simulink model "three_phase_voltage_drop_with_compensation"  (R2024a)
settings: Solver=VariableStepAuto  StartTime=0.0  StopTime=0.4  RelTol=1e-3
undefined symbols (not defined in the file): f, L_line, Q_cap, R_line, V_ll
libraries: dspstat3 x3, spsThreePhaseVIMeasurementLib x2, spsPower3phInstantaneousLib x1, spsThreePhaseParallelRLCLoadLib x1, spsThreePhaseSeriesRLCBranchLib x1, spsThreePhaseSeriesRLCLoadLib x1, spsThreePhaseSourceLib x1, spspowerguiLib x1
settings Model: Creator=m2  LastModifiedBy=m2

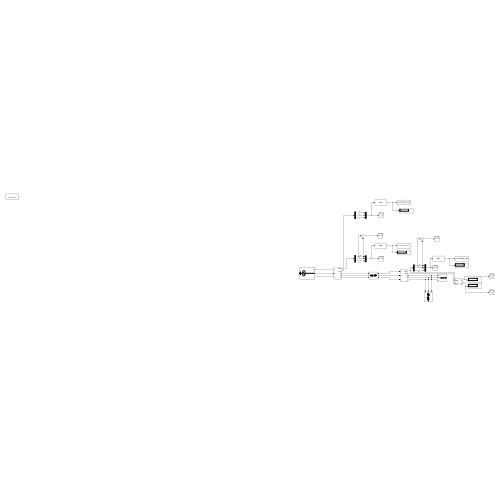
[thumbnail: Simulink's stored preview of the top-level diagram]
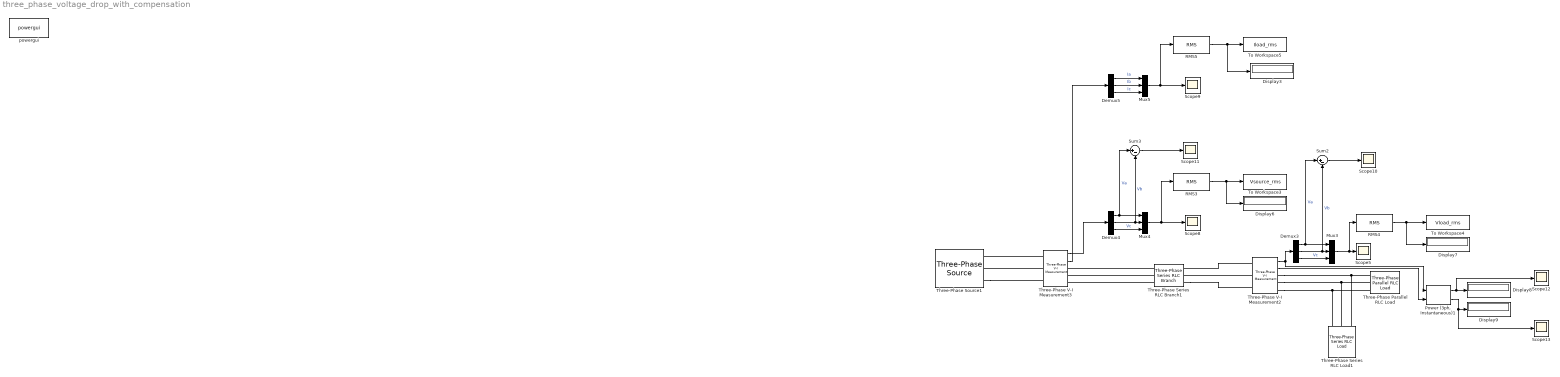
== system three_phase_voltage_drop_with_compensation ==
  Demux3 : Demux  Outputs=3
  Demux4 : Demux  Outputs=3
  Demux5 : Demux  Outputs=3
  Display{3,6..9} (5 alike) : Display
  Mux3 : Mux  Inputs=3
  Mux4 : Mux  Inputs=3
  Mux5 : Mux  Inputs=3
  "Power (3ph, Instantaneous)1" : spsPower3phInstantaneousLib/Power (3ph, Instantaneous)
  RMS3 : dspstat3/RMS  run=off  directionMode=Each column  dimension=1  InputProcessing=Columns as channels (frame based)  reset_popup=None
  RMS4 : dspstat3/RMS  run=off  directionMode=Each column  dimension=1  InputProcessing=Columns as channels (frame based)  reset_popup=None
  RMS5 : dspstat3/RMS  run=off  directionMode=Each column  dimension=1  InputProcessing=Columns as channels (frame based)  reset_popup=None
  Scope{5,8..13} (7 alike) : Scope
  Sum2 : Sum  Inputs=|+-
  Sum3 : Sum  Inputs=|+-
  Three-Phase Parallel RLC Load : spsThreePhaseParallelRLCLoadLib/Three-Phase Parallel RLC Load  LConnTagsString=A|B|C  Configuration=Y (grounded)  NominalVoltage=V_ll  Vabc=[1e3 1e3 1e3]  Vabcp=[1e3 1e3 1e3]  NominalFrequency=f  UnbalancedPower=off  ActivePower=0  InductivePower=0  CapacitivePower=-Q_cap  Pabc=[10e3 9e3 11e3]  QLabc=[100 90 110]  QCabc=[100 90 110]  Pabcp=[10e3 9e3 11e3]  QLabcp=[100 90 110]  QCabcp=[100 90 110]  Measurements=None  LoadType=constant Z
  Three-Phase Series RLC Branch1 : spsThreePhaseSeriesRLCBranchLib/Three-Phase Series RLC Branch  LConnTagsString=A|B|C  RConnTagsString=A|B|C  BranchType=RL  Resistance=R_line  Inductance=L_line  Capacitance=1e-6  Measurements=None
  Three-Phase Series RLC Load1 : spsThreePhaseSeriesRLCLoadLib/Three-Phase Series RLC Load  LConnTagsString=A|B|C  Configuration=Y (grounded)  NominalVoltage=400  Vabc=[1e3 1e3 1e3]  Vabcp=[1e3 1e3 1e3]  NominalFrequency=f  UnbalancedPower=off  ActivePower=P_load  InductivePower=Q_load  CapacitivePower=0  Pabc=[10e3 9e3 11e3]  QLabc=[100 90 110]  QCabc=[100 90 110]  Pabcp=[10e3 9e3 11e3]  QLabcp=[100 90 110]  QCabcp=[100 90 110]  Measurements=None  LoadType=constant Z
  Three-Phase V-I Measurement2 : spsThreePhaseVIMeasurementLib/Three-Phase V-I Measurement  VoltageMeasurement=phase-to-ground  SetLabelV=off  LabelV=Vabc  Vpu=off  VpuLL=off  CurrentMeasurement=yes  SetLabelI=off  LabelI=Iabc  Ipu=off  Pbase=100e6  Vbase=500e3  OutputType=Complex  PhasorSimulation=off  PSBequivalent=0
  Three-Phase V-I Measurement3 : spsThreePhaseVIMeasurementLib/Three-Phase V-I Measurement  VoltageMeasurement=phase-to-ground  SetLabelV=off  LabelV=Vabc  Vpu=off  VpuLL=off  CurrentMeasurement=yes  SetLabelI=off  LabelI=Iabc  Ipu=off  Pbase=100e6  Vbase=500e3  OutputType=Complex  PhasorSimulation=off  PSBequivalent=0
  Three-Phase Source1 : spsThreePhaseSourceLib/Three-Phase Source  InternalConnection=Yg  VoltagePhases=off  Voltage=V_ll  PhaseAngle=0  Voltage_phases=[25e3 25e3 25e3]/sqrt(3)  PhaseAngles_phases=[0 -120 +120]  Frequency=f  NonIdealSource=off  SpecifyImpedance=off  Resistance=0.8929  Inductance=16.58e-3  ShortCircuitLevel=100e6  BaseVoltage=25e3  XRratio=7  BusType=swing  Pref=10e3  Qref=0  Prefabc=[10e3, 10e3, 10e3]  Qrefabc=[0, 0, 0]  Qmin=-inf  Qmax=inf
  To Workspace3 : ToWorkspace  VariableName=Vsource_rms  SaveFormat=Timeseries  SampleTime=-1
  To Workspace4 : ToWorkspace  VariableName=Vload_rms  SaveFormat=Timeseries  SampleTime=-1
  To Workspace5 : ToWorkspace  VariableName=Iload_rms  SaveFormat=Timeseries  SampleTime=-1
  powergui : spspowerguiLib/powergui  Priority=1  SimulationMode=Continuous  SampleTime=50e-6  frequency=60  Iterations=50  frequencyindice=50  Pbase=100e6  ErrMax=1e-4  UnitsV=kV  UnitsW=MW  buscounter=0  FunctionMessages=off  echomessages=off  EnableUseOfTLC=off  CurrentSourceSwitches=off  DisableSnubberDevices=off  DisableRonSwitches=off  DisableVfSwitches=off  DisplayEquations=off  AutomaticDiscreteSolvers=off  SolverType=Tustin/Backward Euler (TBE)  Interpol=off  ExternalGateDelay=off  methode=off  Ts=100  x0status=blocks  SPID=on  SwTol=0  HookPort=off  NonlinearTolerance=1e-4  nMaxIteration=100  ContinueOnMaxIteration=off  RestoreLinks=warning  ResistiveCurrentMeasurement=off  Frange=[0:2:500]  Ylog=off  Xlog=on  ShowGrid=off  save=off  variable=ZData  structure=0  ZoomFFT=off  StartTime=0.0  cycles=1  DisplayStyle=1  fundamental=60  FreqAxis=off  MaxFrequency=1000  frequencyindicesteady=1  RmsSteady=1  display=off
  wires:
  Sum2/1 -> Scope10/1
  RMS5/1 -> Display3/1, To Workspace5/1
  Demux4/1 -> Sum3/1, Mux4/1  "Va"
  Demux4/2 -> Sum3/2, Mux4/2  "Vb"
  Three-Phase V-I Measurement2/2 -> "Power (3ph, Instantaneous)1"/2
  "Power (3ph, Instantaneous)1"/2 -> Scope13/1, Display9/1
  Demux5/3 -> Mux5/3  "Ic"
  RMS4/1 -> To Workspace4/1, Display7/1
  Mux5/1 -> RMS5/1, Scope9/1
  Mux4/1 -> RMS3/1, Scope8/1
  Three-Phase V-I Measurement3/1 -> Demux4/1
  Three-Phase V-I Measurement3/2 -> Demux5/1
  Demux3/3 -> Mux3/3  "Vc"
  Demux5/1 -> Mux5/1  "Ia"
  Demux3/2 -> Sum2/2, Mux3/2  "Vb"
  "Power (3ph, Instantaneous)1"/1 -> Scope12/1, Display8/1
  Demux4/3 -> Mux4/3  "Vc"
  RMS3/1 -> Display6/1, To Workspace3/1
  Mux3/1 -> RMS4/1, Scope5/1
  Three-Phase V-I Measurement2/1 -> "Power (3ph, Instantaneous)1"/1, Demux3/1
  Demux5/2 -> Mux5/2  "Ib"
  Sum3/1 -> Scope11/1
  Demux3/1 -> Sum2/1, Mux3/1  "Va"
  connections:
  Three-Phase Series RLC Branch1/LConn2 -- Three-Phase V-I Measurement3/RConn2
  Three-Phase V-I Measurement2/RConn1 -- Three-Phase Parallel RLC Load/LConn1 -- Three-Phase Series RLC Load1/LConn3
  Three-Phase V-I Measurement2/RConn2 -- Three-Phase Series RLC Load1/LConn2 -- Three-Phase Parallel RLC Load/LConn2
  Three-Phase Series RLC Branch1/RConn3 -- Three-Phase V-I Measurement2/LConn3
  Three-Phase V-I Measurement2/LConn1 -- Three-Phase Series RLC Branch1/RConn1
  Three-Phase Series RLC Branch1/LConn1 -- Three-Phase V-I Measurement3/RConn1
  Three-Phase V-I Measurement2/LConn2 -- Three-Phase Series RLC Branch1/RConn2
  Three-Phase V-I Measurement3/LConn1 -- Three-Phase Source1/RConn1
  Three-Phase Series RLC Branch1/LConn3 -- Three-Phase V-I Measurement3/RConn3
  Three-Phase V-I Measurement2/RConn3 -- Three-Phase Parallel RLC Load/LConn3 -- Three-Phase Series RLC Load1/LConn1
  Three-Phase Source1/RConn3 -- Three-Phase V-I Measurement3/LConn3
  Three-Phase V-I Measurement3/LConn2 -- Three-Phase Source1/RConn2
